simulink library "dspmtrx3"  (Simulink 8.0)
settings: Solver=ode45  SolverMode=SingleTasking  StartTime=0.0  StopTime=10.0  RelTol=1e-3
values from neighbouring files (symbols this model uses):
  a = ver('dsp')    [aboutdspsystbx.m]    (also in dsparch3Transform.m = localGetVal(inData.InstanceData, 'den', '1'); dspddes3Transform.m = sprintf('getYuleWalkerIIRFilterDesignOutput(; dspfdes.m = []; dsprprim.m = a-Mi)
  D = D + B    [rebuffer_delay.m]
undefined symbols (not defined in the file or in its folder): Floor
libraries: dspmtrx3 x5, dspsolvers x3, dspsigattribs x2, dspobslib x1, dspstat3 x1, dspfactors x1
(part 1 of 2)
settings Model: RequirementInfo=9  FPTRunName=Active  Creator=szlotkin  LastModifiedBy=lij  CovMetricSettings=d  ExtModeAutoUpdateStatusClock=off
settings Model: ForwardingTableString=|
  | ||__slOldName__||dspmtrx3/Matrix
  | Sum||__slNewName__||dspobslib/Matrix
  | Sum||__slOldName__||dspmtrx3/Matrix
  | Scaling||__slNewName__||dspmtrx3/Array-Vector
  | Multiply

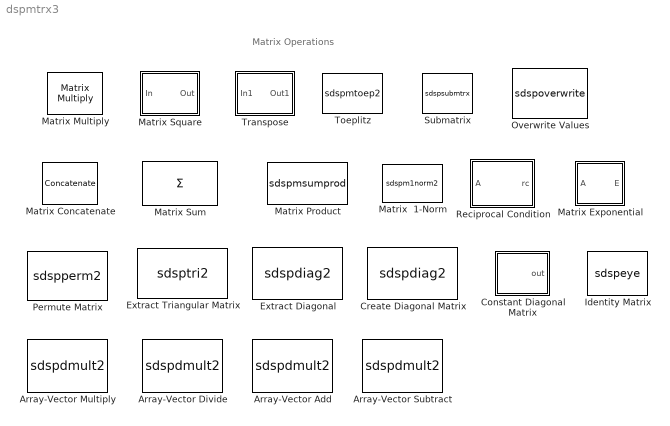
== system dspmtrx3 ==
  note: Matrix Operations
  Array-Vector Add : S-Function  DialogController=dspDDGCreate  DialogControllerArgs=DataTag0  FunctionName=sdspdmult2  Parameters=3,Dimension,V_Source,V_VectFromMask,firstCoeffMin,firstCoeffMax,outputMin,outputMax,dtInfo.firstCoeffMode,dtInfo.firstCoeffWordLength,dtInfo.firstCoeffFracLength,5,0,0,dtInfo.accumMode,dtInfo.accumWordLength,dtInfo.accumFracLength,dtInfo.outputMode,dtInfo.outputWordLength,dtInfo.outputFracLength,dtInfo.roundingMode,dtInfo.overflowMode  EnableBusSupport=off  mask(Array-Vector Add){Dimension=1, V_Source=Input port, V_VectFromMask=[0.5 0.25], additionalParams=off, allowOverrides=on, firstCoeffMode=Same word length as input, firstCoeffSignedness=Auto, firstCoeffWordLength=16, firstCoeffFracLength=15, firstCoeffDataTypeStr=Inherit: Same word length as input, firstCoeffLastDataTypeStr=Inherit: Same word length as input, firstCoeffMin=[], firstCoeffMax=[], outputMode=Same as accumulator, outputSignedness=Auto, outputWordLength=16, outputFracLength=15, outputDataTypeStr=Inherit: Same as accumulator, outputLastDataTypeStr=Inherit: Same as accumulator, outputMin=[], outputMax=[], accumMode=Inherit via internal rule, accumSignedness=Auto, accumWordLength=32, accumFracLength=30, accumDataTypeStr=Inherit: Inherit via internal rule, accumLastDataTypeStr=Inherit: Inherit via internal rule, prodOutputMode=Inherit via internal rule, prodOutputSignedness=Auto, prodOutputWordLength=32, prodOutputFracLength=30, roundingMode=Floor, overflowMode=off, LockScale=off}
      mask prompts: Dimension "Add along dimension:"; V_Source "Vector (V) source:"; V_VectFromMask "Vector (V):"; additionalParams "------- Show additional parameters -------"; allowOverrides "Allow overrides from DSP Fixed-Point Attributes blocks"; firstCoeffMode "Fixed-point scaling vector attributes:"; firstCoeffSignedness "Scaling vector elements signedness:"; firstCoeffWordLength "Scaling vector elements word length:"; firstCoeffFracLength "Scaling vector elements fraction length:"; firstCoeffDataTypeStr "Vector (V) data type string:"; firstCoeffLastDataTypeStr "Last vector (V) data type string:"; firstCoeffMin "Vector (V) minimum:"; firstCoeffMax "Vector (V) maximum:"; outputMode "Fixed-point output attributes:"; outputSignedness "Output signedness:"; outputWordLength "Output word length:"; outputFracLength "Output fraction length:"; outputDataTypeStr "Output data type string:"; outputLastDataTypeStr "Last output data type string:"; outputMin "Output minimum:"; outputMax "Output maximum:"; accumMode "Fixed-point accumulator attributes:"; accumSignedness "Accumulator signedness:"; accumWordLength "Accumulator word length"; accumFracLength "Accumulator fraction length:"; accumDataTypeStr "Accum data type string:"; accumLastDataTypeStr "Last accum data type string:"; prodOutputMode "Fixed-point product output attributes:"; prodOutputSignedness "Product output signedness:"; prodOutputWordLength "Product output word length:"; prodOutputFracLength "Product output fraction length:"; roundingMode "Round integer calculations toward:"; overflowMode "Saturate on integer overflow"; LockScale "Lock scaling"
      mask help: Add the input array A to the elements of vector V along the specified dimension. Note that unoriented input signals are treated as oriented column vectors. The output of this block is always oriented.
      mask init:
      | blkh   = gcbh;
      | dtRows = dspblkGetArrayVectorAddSubDTRowInfo();
      | dtInfo = dspGetUDTFixptDataTypeInfo(blkh, dtRows, true);
      mask Help: eval('blocksethelp');
      mask StyleString: edit,popup(Input port|Dialog parameter),edit,checkbox,checkbox,popup(Same word length as input|Specify word length|Binary point scaling|Slope and bias scaling|User-defined),popup(Auto|Signed),edit,edit,unidt({a=10|12|13|3}{i=Inherit: Same word length as input}{s=UDTBinaryPointMode}{g=UDTSignedSign}),edit,min,max,popup(Same as accumulator|Same as first input|Binary point scaling|Slope and bias scaling|User-defined),popup(Auto|Signed),edit,edit,unidt({a=18|20|21|}{i=Inherit: Same as first input|Inherit: Same as accumulator}{s=UDTBinaryPointMode}{g=UDTSignedSign|UDTInheritSign}),edit,min,max,popup(Inherit via internal rule|Same as first input|Binary point scaling|Slope and bias scaling|User-defined),popup(Auto|Signed),edit,edit,unidt({a=26|||}{i=Inherit: Inherit via internal rule|Inherit: Same as first input}{s=UDTBinaryPointMode}{g=UDTSignedSign|UDTInheritSign}),edit,popup(Inherit via internal rule|Same as first input|Binary point scaling|Slope and bias scaling|User-defined),popup(Auto|Signed),edit,edit,popup(Ceiling|Convergent|Floor|Nearest|Round|Simplest|Zero),checkbox,checkbox
      mask Display:
      | inp1_index = 1;
      | inp1_label = 'A';
      | if (V_Source == 1),
      |   inp2_index = 2;
      |   inp2_label = 'V';
      | else
      |   inp2_index = 1;
      |   inp2_label = 'A';
      | end
      | 
      | port_label('input',inp1_index,inp1_label);
      | port_label('input',inp2_index,inp2_label);
      | disp('Array-Vector\nAdd');
  Array-Vector Divide : S-Function  DialogController=dspDDGCreate  DialogControllerArgs=DataTag1  FunctionName=sdspdmult2  Parameters=2,Dimension,V_Source,V_VectFromMask,firstCoeffMin,firstCoeffMax,outputMin,outputMax,dtInfo.firstCoeffMode,dtInfo.firstCoeffWordLength,dtInfo.firstCoeffFracLength,5,0,0,5,0,0,dtInfo.outputMode,dtInfo.outputWordLength,dtInfo.outputFracLength,dtInfo.roundingMode,dtInfo.overflowMode  EnableBusSupport=off  mask(Array-Vector Divide){Dimension=1, V_Source=Input port, V_VectFromMask=[0.5 0.25], additionalParams=off, allowOverrides=on, firstCoeffMode=Same word length as input, firstCoeffSignedness=Auto, firstCoeffWordLength=16, firstCoeffFracLength=15, firstCoeffDataTypeStr=Inherit: Same word length as input, firstCoeffLastDataTypeStr=Inherit: Same word length as input, firstCoeffMin=[], firstCoeffMax=[], outputMode=Same as first input, outputSignedness=Auto, outputWordLength=16, outputFracLength=15, outputDataTypeStr=Inherit: Same as first input, outputLastDataTypeStr=Inherit: Same as first input, outputMin=[], outputMax=[], accumMode=Inherit via internal rule, accumSignedness=Auto, accumWordLength=32, accumFracLength=30, prodOutputMode=Inherit via internal rule, prodOutputSignedness=Auto, prodOutputWordLength=32, prodOutputFracLength=30, roundingMode=Floor, overflowMode=off, LockScale=off}
      mask prompts: Dimension "Divide along dimension:"; V_Source "Vector (V) source:"; V_VectFromMask "Vector (V):"; additionalParams "------- Show additional parameters -------"; allowOverrides "Allow overrides from DSP Fixed-Point Attributes blocks"; firstCoeffMode "Fixed-point scaling vector attributes:"; firstCoeffSignedness "Scaling vector elements signedness:"; firstCoeffWordLength "Scaling vector elements word length:"; firstCoeffFracLength "Scaling vector elements fraction length:"; firstCoeffDataTypeStr "Vector (V) data type string:"; firstCoeffLastDataTypeStr "Last vector (V) data type string:"; firstCoeffMin "Vector (V) minimum:"; firstCoeffMax "Vector (V) maximum:"; outputMode "Fixed-point output attributes:"; outputSignedness "Output signedness:"; outputWordLength "Output word length:"; outputFracLength "Output fraction length:"; outputDataTypeStr "Output data type string:"; outputLastDataTypeStr "Last output data type string:"; outputMin "Output minimum:"; outputMax "Output maximum:"; accumMode "Fixed-point accumulator attributes:"; accumSignedness "Accumulator signedness:"; accumWordLength "Accumulator word length"; accumFracLength "Accumulator fraction length:"; prodOutputMode "Fixed-point product output attributes:"; prodOutputSignedness "Product output signedness:"; prodOutputWordLength "Product output word length:"; prodOutputFracLength "Product output fraction length:"; roundingMode "Round integer calculations toward:"; overflowMode "Saturate on integer overflow"; LockScale "Lock scaling"
      mask help: Divide the input array A by the elements of vector V along the specified dimension. In the two-dimensional case, this is equivalent to dividing a full matrix (A) by a diagonal (V). Note that unoriented input signals are treated as oriented column vectors. The output of this block is always oriented.
      mask init:
      | blkh   = gcbh;
      | dtRows = dspblkGetArrayVectorDivDTRowInfo();
      | dtInfo = dspGetUDTFixptDataTypeInfo(blkh, dtRows, true);
      mask Help: eval('blocksethelp');
      mask StyleString: edit,popup(Input port|Dialog parameter),edit,checkbox,checkbox,popup(Same word length as input|Specify word length|Binary point scaling|Slope and bias scaling|User-defined),popup(Auto|Signed),edit,edit,unidt({a=10|12|13|3}{i=Inherit: Same word length as input}{s=UDTBinaryPointMode}{g=UDTSignedSign}),edit,min,max,popup(Same as first input|Binary point scaling|Slope and bias scaling|User-defined),popup(Auto|Signed),edit,edit,unidt({a=18|20|21|}{i=Inherit: Same as first input}{s=UDTBinaryPointMode}{g=UDTSignedSign|UDTInheritSign}),edit,min,max,popup(Inherit via internal rule|Same as product output|Same as first input|Binary point scaling|Slope and bias scaling|User-defined),popup(Auto|Signed),edit,edit,popup(Inherit via internal rule|Same as first input|Binary point scaling|Slope and bias scaling|User-defined),popup(Auto|Signed),edit,edit,popup(Ceiling|Convergent|Floor|Nearest|Round|Simplest|Zero),checkbox,checkbox
      mask Display:
      | inp1_index = 1;
      | inp1_label = 'A';
      | if (V_Source == 1),
      |   inp2_index = 2;
      |   inp2_label = 'V';
      | else
      |   inp2_index = 1;
      |   inp2_label = 'A';
      | end
      | 
      | port_label('input',inp1_index,inp1_label);
      | port_label('input',inp2_index,inp2_label);
      | disp('Array-Vector\nDivide');
  Array-Vector Multiply : S-Function  DialogController=dspDDGCreate  DialogControllerArgs=DataTag2  FunctionName=sdspdmult2  Parameters=1,Dimension,V_Source,V_VectFromMask,firstCoeffMin,firstCoeffMax,outputMin,outputMax,dtInfo.firstCoeffMode,dtInfo.firstCoeffWordLength,dtInfo.firstCoeffFracLength,dtInfo.prodOutputMode,dtInfo.prodOutputWordLength,dtInfo.prodOutputFracLength,dtInfo.accumMode,dtInfo.accumWordLength,dtInfo.accumFracLength,dtInfo.outputMode,dtInfo.outputWordLength,dtInfo.outputFracLength,dtInfo.roundingMode,dtInfo.overflowMode  EnableBusSupport=off  mask(Array-Vector Multiply){mode=Mute, saveAsFlag=0, Dimension=2, V_Source=Input port, V_VectFromMask=[0.5 0.25], additionalParams=off, allowOverrides=on, firstCoeffMode=Same word length as input, firstCoeffSignedness=Auto, firstCoeffWordLength=16, firstCoeffFracLength=15, firstCoeffDataTypeStr=Inherit: Same word length as input, firstCoeffLastDataTypeStr=Inherit: Same word length as input, firstCoeffMin=[], firstCoeffMax=[], outputMode=Same as product output, outputSignedness=Auto, outputWordLength=16, outputFracLength=15, outputDataTypeStr=Inherit: Same as product output, outputLastDataTypeStr=Inherit: Same as product output, outputMin=[], outputMax=[], accumMode=Inherit via internal rule, accumSignedness=Auto, accumWordLength=32, accumFracLength=30, accumDataTypeStr=Inherit: Inherit via internal rule, accumLastDataTypeStr=Inherit: Inherit via internal rule, prodOutputMode=Inherit via internal rule, prodOutputSignedness=Auto, prodOutputWordLength=32, prodOutputFracLength=30, prodOutputDataTypeStr=Inherit: Inherit via internal rule, prodOutputLastDataTypeStr=Inherit: Inherit via internal rule, roundingMode=Floor, overflowMode=off, LockScale=off}
      mask prompts: saveAsFlag "Save_as flag:"; Dimension "Multiply along dimension:"; V_Source "Vector (V) source:"; V_VectFromMask "Vector (V):"; additionalParams "------- Show additional parameters -------"; allowOverrides "Allow overrides from DSP Fixed-Point Attributes blocks"; firstCoeffMode "Fixed-point scaling vector attributes:"; firstCoeffSignedness "Scaling vector elements signedness:"; firstCoeffWordLength "Scaling vector elements word length:"; firstCoeffFracLength "Scaling vector elements fraction length:"; firstCoeffDataTypeStr "Vector (V) data type string:"; firstCoeffLastDataTypeStr "Last vector (V) data type string:"; firstCoeffMin "Last vector (V) minimum:"; firstCoeffMax "Last vector (V) maximum:"; outputMode "Fixed-point output attributes:"; outputSignedness "Output signedness:"; outputWordLength "Output word length:"; outputFracLength "Output fraction length:"; outputDataTypeStr "Output data type string:"; outputLastDataTypeStr "Last output data type string:"; outputMin "Output minimum:"; outputMax "Output maximum:"; accumMode "Fixed-point accumulator attributes:"; accumSignedness "Accumulator signedness:"; accumWordLength "Accumulator word length"; accumFracLength "Accumulator fraction length:"; accumDataTypeStr "Accum data type string:"; accumLastDataTypeStr "Last accum data type string:"; prodOutputMode "Fixed-point product output attributes:"; prodOutputSignedness "Product output signedness:"; prodOutputWordLength "Product output word length:"; prodOutputFracLength "Product output fraction length:"; prodOutputDataTypeStr "ProdOutput data type string:"; prodOutputLastDataTypeStr "Last prodOutput data type string:"; roundingMode "Round integer calculations toward:"; overflowMode "Saturate on integer overflow"; LockScale "Lock scaling"
      mask help: Multiply the input array A by the elements of vector V along the specified dimension. In the two-dimensional case, this is equivalent to multiplying a full matrix (A) by a diagonal (V). Note that unoriented input signals are treated as oriented column vectors. The output of this block is always oriented.
      mask init:
      | blkh = gcbh;
      | m    = get_param(blkh, 'mode');
      | if (~strcmp(m, 'Mute'))
      |     if (saveAsFlag == 0)
      |         if strcmp(m,'Scale rows (D*A)')
      |             set_param(blkh, 'Dimension', '1', 'mode', 'Mute');
      |         elseif strcmp(m,'Scale columns (A*D)')
      |             set_param(blkh, 'Dimension', '2', 'mode', 'Mute');
      |         end
      |     end
      | end
      | dtRows = dspblkGetArrayVectorMpyDTRowInfo();
      | dtInfo = dspGetUDTFixptDataTypeInfo(blkh, dtRows, true);
      mask Help: eval('blocksethelp');
      mask StyleString: popup(Scale rows (D*A)|Scale columns (A*D)|Mute),edit,edit,popup(Input port|Dialog parameter),edit,checkbox,checkbox,popup(Same word length as input|Specify word length|Binary point scaling|Slope and bias scaling|User-defined),popup(Auto|Signed),edit,edit,unidt({a=12|14|15|5}{i=Inherit: Same word length as input}{s=UDTBinaryPointMode}{g=UDTSignedSign}),edit,min,max,popup(Same as product output|Same as first input|Binary point scaling|Slope and bias scaling|User-defined),popup(Auto|Signed),edit,edit,unidt({a=20|22|23|}{i=Inherit: Same as first input|Inherit: Same as product output}{s=UDTBinaryPointMode}{g=UDTSignedSign|UDTInheritSign}),edit,min,max,popup(Inherit via internal rule|Same as product output|Same as first input|Binary point scaling|Slope and bias scaling|User-defined),popup(Auto|Signed),edit,edit,unidt({a=28|||}{i=Inherit: Inherit via internal rule|Inherit: Same as first input|Inherit: Same as product output}{s=UDTBinaryPointMode}{g=UDTSignedSign|UDTInheritSign}),edit,popup(Inherit via internal rule|Same as first input|Binary point scaling|Slope and bias scaling|User-defined),popup(Auto|Signed),edit,edit,unidt({a=34|||}{i=Inherit: Inherit via internal rule|Inherit: Same as first input}{s=UDTBinaryPointMode}{g=UDTSignedSign|UDTInheritSign}),edit,popup(Ceiling|Convergent|Floor|Nearest|Round|Simplest|Zero),checkbox,checkbox
      mask Display:
      | inp1_index = 1;
      | inp1_label = 'A';
      | if (V_Source == 1),
      |   inp2_index = 2;
      |   inp2_label = 'V';
      | else
      |   inp2_index = 1;
      |   inp2_label = 'A';
      | end
      | 
      | port_label('input',inp1_index,inp1_label);
      | port_label('input',inp2_index,inp2_label);
      | disp('Array-Vector\nMultiply');
  Array-Vector Subtract : S-Function  DialogController=dspDDGCreate  DialogControllerArgs=DataTag3  FunctionName=sdspdmult2  Parameters=4,Dimension,V_Source,V_VectFromMask,firstCoeffMin,firstCoeffMax,outputMin,outputMax,dtInfo.firstCoeffMode,dtInfo.firstCoeffWordLength,dtInfo.firstCoeffFracLength,5,0,0,dtInfo.accumMode,dtInfo.accumWordLength,dtInfo.accumFracLength,dtInfo.outputMode,dtInfo.outputWordLength,dtInfo.outputFracLength,dtInfo.roundingMode,dtInfo.overflowMode  EnableBusSupport=off  mask(Array-Vector Subtract){Dimension=1, V_Source=Input port, V_VectFromMask=[0.5 0.25], additionalParams=off, allowOverrides=on, firstCoeffMode=Same word length as input, firstCoeffSignedness=Auto, firstCoeffWordLength=16, firstCoeffFracLength=15, firstCoeffDataTypeStr=Inherit: Same word length as input, firstCoeffLastDataTypeStr=Inherit: Same word length as input, firstCoeffMin=[], firstCoeffMax=[], outputMode=Same as accumulator, outputSignedness=Auto, outputWordLength=16, outputFracLength=15, outputDataTypeStr=Inherit: Same as accumulator, outputLastDataTypeStr=Inherit: Same as accumulator, outputMin=[], outputMax=[], accumMode=Inherit via internal rule, accumSignedness=Auto, accumWordLength=32, accumFracLength=30, accumDataTypeStr=Inherit: Inherit via internal rule, accumLastDataTypeStr=Inherit: Inherit via internal rule, prodOutputMode=Inherit via internal rule, prodOutputSignedness=Auto, prodOutputWordLength=32, prodOutputFracLength=30, roundingMode=Floor, overflowMode=off, LockScale=off}
      mask prompts: Dimension "Subtract along dimension:"; V_Source "Vector (V) source:"; V_VectFromMask "Vector (V):"; additionalParams "------- Show additional parameters -------"; allowOverrides "Allow overrides from DSP Fixed-Point Attributes blocks"; firstCoeffMode "Fixed-point scaling vector attributes:"; firstCoeffSignedness "Scaling vector elements signedness:"; firstCoeffWordLength "Scaling vector elements word length:"; firstCoeffFracLength "Scaling vector elements fraction length:"; firstCoeffDataTypeStr "Vector (V) data type string:"; firstCoeffLastDataTypeStr "Last vector (V) data type string:"; firstCoeffMin "Vector (V) minimum:"; firstCoeffMax "Vector (V) maximum:"; outputMode "Fixed-point output attributes:"; outputSignedness "Output signedness:"; outputWordLength "Output word length:"; outputFracLength "Output fraction length:"; outputDataTypeStr "Output data type string:"; outputLastDataTypeStr "Last output data type string:"; outputMin "Output minimum:"; outputMax "Output maximum:"; accumMode "Fixed-point accumulator attributes:"; accumSignedness "Accumulator signedness:"; accumWordLength "Accumulator word length"; accumFracLength "Accumulator fraction length:"; accumDataTypeStr "Accum data type string:"; accumLastDataTypeStr "Last accum data type string:"; prodOutputMode "Fixed-point product output attributes:"; prodOutputSignedness "Product output signedness:"; prodOutputWordLength "Product output word length:"; prodOutputFracLength "Product output fraction length:"; roundingMode "Round integer calculations toward:"; overflowMode "Saturate on integer overflow"; LockScale "Lock scaling"
      mask help: Subtract the elements of vector V from input array A along the specified dimension. Note that unoriented input signals are treated as oriented column vectors. The output of this block is always oriented.
      mask init:
      | blkh   = gcbh;
      | dtRows = dspblkGetArrayVectorAddSubDTRowInfo();
      | dtInfo = dspGetUDTFixptDataTypeInfo(blkh, dtRows, true);
      mask Help: eval('blocksethelp');
      mask StyleString: edit,popup(Input port|Dialog parameter),edit,checkbox,checkbox,popup(Same word length as input|Specify word length|Binary point scaling|Slope and bias scaling|User-defined),popup(Auto|Signed),edit,edit,unidt({a=10|12|13|3}{i=Inherit: Same word length as input}{s=UDTBinaryPointMode}{g=UDTSignedSign}),edit,min,max,popup(Same as accumulator|Same as first input|Binary point scaling|Slope and bias scaling|User-defined),popup(Auto|Signed),edit,edit,unidt({a=18|20|21|}{i=Inherit: Same as first input|Inherit: Same as accumulator}{s=UDTBinaryPointMode}{g=UDTSignedSign|UDTInheritSign}),edit,min,max,popup(Inherit via internal rule|Same as first input|Binary point scaling|Slope and bias scaling|User-defined),popup(Auto|Signed),edit,edit,unidt({a=26|||}{i=Inherit: Inherit via internal rule|Inherit: Same as first input}{s=UDTBinaryPointMode}{g=UDTSignedSign|UDTInheritSign}),edit,popup(Inherit via internal rule|Same as first input|Binary point scaling|Slope and bias scaling|User-defined),popup(Auto|Signed),edit,edit,popup(Ceiling|Convergent|Floor|Nearest|Round|Simplest|Zero),checkbox,checkbox
      mask Display:
      | inp1_index = 1;
      | inp1_label = 'A';
      | if (V_Source == 1),
      |   inp2_index = 2;
      |   inp2_label = 'V';
      | else
      |   inp2_index = 1;
      |   inp2_label = 'A';
      | end
      | 
      | port_label('input',inp1_index,inp1_label);
      | port_label('input',inp2_index,inp2_label);
      | disp('Array-Vector\nSubtract');
  Constant Diagonal Matrix : Subsystem  mask(Constant Diagonal Matrix){q=ones(1,3), frame=off, additionalParams=off, allowOverrides=on, dataType=Inherit from 'Constant(s) along diagonal', isSigned=on, wordLen=16, udDataType=sfix(16), fracBitsMode=Best precision, numFracBits=15}
      mask prompts: q "Constant(s) along diagonal:"; frame "Frame-based output"; additionalParams "------- Show additional parameters --------"; allowOverrides "Allow overrides by DSP Fixed-Point Attributes blocks"; dataType "Output data type:"; isSigned "Signed"; wordLen "Word length:"; udDataType "User-defined data type:"; fracBitsMode "Set fraction length in output to:"; numFracBits "Fraction length:"
      mask help: Generate a diagonal matrix having elements specified by a vector constant.
      mask init:
      | [a,x,y] = dspblkconstdiag('icon',q);
      | dspblkconstdiag('init');
      mask Help: eval('blocksethelp');
      mask StyleString: edit,checkbox,checkbox,checkbox,popup(double|single|int8|uint8|int16|uint16|int32|uint32|boolean|Fixed-point|User-defined|Inherit from 'Constant(s) along diagonal'|Inherit via back propagation),checkbox,edit,edit,popup(Best precision|User-defined),edit
      mask CallbackString: ||||dspblkconstdiag;|||dspblkconstdiag;|dspblkconstdiag;|
      mask TabNameString: Main,Main,Main,Main,Data Types,Data Types,Data Types,Data Types,Data Types,Data Types
      mask Display: plot(x,y)
  Create Diagonal Matrix : S-Function  FunctionName=sdspdiag2  Parameters=mode  EnableBusSupport=off  mask(Create Diagonal Matrix){}
      mask help: Convert a vector of diagonal elements to a full matrix.
      mask init:
      | mode = 1;
      | x = [.58 .87 .87 .58 .58 NaN 0.45 0.12 NaN 0.525 0.525 0.475 0.475 0.525 0.525 0.565 0.525 ];
      | y = [ 0.2 0.2 0.8 0.8 0.2 NaN 0.2 0.8 NaN 0.435 0.475 0.475 0.525 0.525 0.565 0.5 0.435 ];
      mask Help: eval('blocksethelp');
      mask Display:
      | plot(x,y);
      | port_label('input',1,'D');
      | port_label('output',1,'A');
  Extract Diagonal : S-Function  FunctionName=sdspdiag2  Parameters=mode  EnableBusSupport=off  mask(Extract Diagonal){}
      mask help: Extract the main diagonal of a full matrix.
      mask init:
      | mode = 2;
      | x = [.58 .87 NaN 0.12 0.45 0.45 0.12 0.12 NaN 0.525 0.525 0.475 0.475 0.525 0.525 0.565 0.525 ];
      | y = [ 0.8 0.2 NaN 0.2 0.2 0.8 0.8 0.2 NaN 0.435 0.475 0.475 0.525 0.525 0.565 0.5 0.435 ];
      mask Help: eval('blocksethelp');
      mask Display:
      | plot(x,y);
      | port_label('input',1,'A');
      | port_label('output',1,'D');
  Extract Triangular Matrix : S-Function  FunctionName=sdsptri2  Parameters=fcn  EnableBusSupport=off  mask(Extract Triangular Matrix){fcn=Upper}
      mask prompts: fcn "Extract:"
      mask help: Extract upper or lower triangular part of input matrix.
      mask init:
      | [s,x,y] = dspblktri(fcn);
      mask Help: eval('blocksethelp');
      mask StyleString: popup(Upper|Lower)
      mask Display:
      | plot(x,y);
      | port_label('input',1,'A');
      | port_label('output',1,s);
  Identity Matrix : S-Function  FunctionName=sdspeye  Parameters=Inherit,N,Ts,isCustomFloat,fxpIsSigned,dTypeID,fxpWordLength,fxpFracLength,1  EnableBusSupport=off  mask(Identity Matrix){Inherit=off, N=5, Ts=1, additionalParams=off, allowOverrides=on, dataType=double, isSigned=on, wordLen=16, udDataType=sfix(16), fracBitsMode=Best precision, numFracBits=15, OutDataTypeStr=double, LastOutDataTypeStr=double}
      mask prompts: Inherit "Inherit output port attributes from input port"; N "Matrix size:"; Ts "Sample time:"; additionalParams "------- Show additional parameters --------"; allowOverrides "Allow overrides by DSP Fixed-Point Attributes blocks"; dataType "Output data type:"; isSigned "Signed"; wordLen "Word length:"; udDataType "User-defined data type (e.g. sfix(16), float('single')):"; fracBitsMode "Set fraction length in output to:"; numFracBits "Fraction length:"; OutDataTypeStr "Output data type:"; LastOutDataTypeStr "Last output data type:"
      mask help: Output an identity matrix. If the matrix size entered is a scalar, then the output will be a square (symmetric) identity matrix with the number of rows and columns both equal to the specified value. If the matrix size entered is a two-element vector [M N], then the output will be an asymmetric matrix with the number of rows equal to M, the number of columns equal to N, ones down the diagonal, and zeros elsewhere. This matches the syntax of the MATLAB function eye(N) and eye(M,N), respectively.
      mask init:
      | isCustomFloat =  0; % nice default
      | fxpIsSigned   =  1; % nice default
      | fxpWordLength =  8; % nice default
      | fxpFracLength =  0; % nice default
      | if Inherit
      |     dTypeID   = -3; % SAME_AS_INPUT
      | else
      |     dtRows            = dspblkGetDiscreteImpulseDTRowInfo();
      |     [dtInfo, dTypeID] = dspblkUDTMapperOutDType(gcbh, dtRows{1}, 'dataType', 1.0);
      |     isCustomFloat     = dtInfo.DataTypeIsCustomFloat;
      |     if ~isCustomFloat
      |         fxpIsSigned   = dtInfo.DataTypeIsSigned;
      |         fxpWordLength = dtInfo.DataTypeWordLength;
      |         fxpFracLength = dtInfo.DataTypeFracOrMantBits;
      |     end
      | end
      mask Help: eval('blocksethelp');
      mask StyleString: checkbox,edit,edit,checkbox,checkbox,popup(double|single|int8|uint8|int16|uint16|int32|uint32|boolean|Fixed-point|User-defined|Inherit via back propagation),checkbox,edit,edit,popup(Best precision|User-defined),edit,unidt({a=12|||}{i=Inherit: Inherit via back propagation}{b=double|single|int8|uint8|int16|uint16|int32|uint32|boolean}{s=UDTBinaryPointMode|UDTBestPrecisionMode}{g=UDTSignedSign|UDTUnsignedSign}),edit
      mask CallbackString: dspblkeye||||||||||||
      mask TabNameString: Main,Main,Main,Data Types,Data Types,Data Types,Data Types,Data Types,Data Types,Data Types,Data Types,Data Types,Data Types
      mask Display:
      | if Inherit
      |     disp('eye( )');
      | else
      |     disp(['eye(' , num2str(get_param(gcbh, 'N')), ')']);
      | end
  Matrix Concatenate : Concatenate  Mode=Multidimensional array  ConcatenateDimension=2
  Matrix Exponential : Subsystem
      mask Type: Matrix Exponential
      mask Description: Compute the matrix exponential, using a scaling and squaring algorithm with a Pade approximation.  Matrix must be square.
      mask Help: eval('blocksethelp');
      mask Display: disp('expm')
  Matrix Product : S-Function  DialogController=dspDDGCreate  DialogControllerArgs=DataTag4  FunctionName=sdspmsumprod  Parameters=Dim,2,outputMin,outputMax,dtInfo.interProdMode,dtInfo.interProdWordLength,dtInfo.interProdFracLength,dtInfo.prodOutputMode,dtInfo.prodOutputWordLength,dtInfo.prodOutputFracLength,dtInfo.accumMode,dtInfo.accumWordLength,dtInfo.accumFracLength,dtInfo.outputMode,dtInfo.outputWordLength,dtInfo.outputFracLength,dtInfo.roundingMode,dtInfo.overflowMode  EnableBusSupport=off  mask(Matrix Product){Dim=Columns, additionalParams=off, allowOverrides=on, outputMode=Same as product output, outputWordLength=16, outputFracLength=15, outputDataTypeStr=Inherit: Same as product output, outputLastDataTypeStr=Inherit: Same as product output, outputMin=[], outputMax=[], accumMode=Inherit via internal rule, accumWordLength=32, accumFracLength=30, accumDataTypeStr=Inherit: Inherit via internal rule, accumLastDataTypeStr=Inherit: Inherit via internal rule, prodOutputMode=Inherit via internal rule, prodOutputWordLength=32, prodOutputFracLength=30, prodOutputDataTypeStr=Inherit: Inherit via internal rule, prodOutputLastDataTypeStr=Inherit: Inherit via internal rule, interProdMode=Same as input, interProdWordLength=16, interProdFracLength=15, interProdDataTypeStr=Inherit: Same as input, interProdLastDataTypeStr=Inherit: Same as input, roundingMode=Floor, overflowMode=off, LockScale=off}
      mask prompts: Dim "Multiply over:"; additionalParams "------- Show additional parameters -------"; allowOverrides "Allow overrides from DSP Fixed-Point Attributes blocks"; outputMode "Fixed-point output attributes:"; outputWordLength "Output word length:"; outputFracLength "Output fraction length:"; outputDataTypeStr "Output data type string:"; outputLastDataTypeStr "Last output data type string:"; outputMin "Output minimum:"; outputMax "Output maximum:"; accumMode "Fixed-point accumulator attributes:"; accumWordLength "Accumulator word length:"; accumFracLength "Accumulator fraction length:"; accumDataTypeStr "Accum data type string:"; accumLastDataTypeStr "Last accum data type string:"; prodOutputMode "Fixed-point product output attributes:"; prodOutputWordLength "Product output word length:"; prodOutputFracLength "Product output fraction length:"; prodOutputDataTypeStr "ProdOutput data type string:"; prodOutputLastDataTypeStr "Last prodOutput data type string:"; interProdMode "Fixed-point intermediate product attributes:"; interProdWordLength "Intermediate product word length:"; interProdFracLength "Intermediate product fraction length:"; interProdDataTypeStr "Intermediate product data type string:"; interProdLastDataTypeStr "Last intermediate product data type string:"; roundingMode "Round integer calculations toward:"; overflowMode "Saturate on integer overflow"; LockScale "Lock scaling"
      mask help: Multiply the elements of a matrix along its rows, its columns, or over all its elements. Note that 1-D input signals produce a single scalar output equal to the product of the individual elements.
      mask init:
      | blkh   = gcbh;
      | dtRows = dspblkGetMtrxProdDTRowInfo();
      | dtInfo = dspGetUDTFixptDataTypeInfo(blkh, dtRows, true);
      mask Help: eval('blocksethelp');
      mask StyleString: popup(Rows|Columns|Entire input),checkbox,checkbox,popup(Same as product output|Same as input|Binary point scaling|Slope and bias scaling|User-defined),edit,edit,unidt({a=7|9|10|}{i=Inherit: Same as input|Inherit: Same as product output}{s=UDTBinaryPointMode}{g=UDTInheritSign}),edit,min,max,popup(Inherit via internal rule|Same as product output|Same as input|Binary point scaling|Slope and bias scaling|User-defined),edit,edit,unidt({a=14|||}{i=Inherit: Inherit via internal rule|Inherit: Same as input|Inherit: Same as product output}{s=UDTBinaryPointMode}{g=UDTInheritSign}),edit,popup(Inherit via internal rule|Same as input|Binary point scaling|Slope and bias scaling|User-defined),edit,edit,unidt({a=19|||}{i=Inherit: Inherit via internal rule|Inherit: Same as input}{s=UDTBinaryPointMode}{g=UDTInheritSign}),edit,popup(Same as input|Binary point scaling|Slope and bias scaling|User-defined),edit,edit,unidt({a=24|||}{i=Inherit: Same as input}{s=UDTBinaryPointMode}{g=UDTInheritSign}),edit,popup(Ceiling|Convergent|Floor|Nearest|Round|Simplest|Zero),checkbox,checkbox
      mask Display:
      | if (Dim==1), str='Row\nProduct';
      | elseif (Dim==2), str='Column\nProduct';
      | else str='Product of\nAll Elements';
      | end
      | disp(str);
  Matrix Square : Subsystem  mask(Matrix Square){OutMin=[], OutMax=[], OutDataTypeStr=Inherit: Inherit via internal rule, LockScale=off, RndMeth=Floor, SaturateOnIntegerOverflow=off}
      mask prompts: OutMin "Output minimum:"; OutMax "Output maximum:"; OutDataTypeStr "Output data type:"; LockScale "Lock output data type setting against changes by the fixed-point tools"; RndMeth "Integer rounding mode:"; SaturateOnIntegerOverflow "Saturate on integer overflow"
      mask help: Compute the matrix square, U' * U. Hermitian transpose is performed for complex inputs. [Mx1] and [1xN] input matrices may be used to compute efficient outer and inner products, respectively.
      mask init:
      | mtxsqName = gcb;
      | trnspName = sprintf('%s/Math\nFunction', mtxsqName);
      | prdctName = sprintf('%s/Product', mtxsqName);
      | % Set matrix transpose block parameters
      | set_param(trnspName, 'SaturateOnIntegerOverflow', SaturateOnIntegerOverflow);
      | % Set matrix product block parameters
      | set_param(prdctName, 'SaturateOnIntegerOverflow', SaturateOnIntegerOverflow);
      | switch RndMeth
      |     case 1
      |         set_param(prdctName, 'RndMeth', 'Ceiling');
      |     case 2
      |         set_param(prdctName, 'RndMeth', 'Convergent');
      |     case 3
      |         set_param(prdctName, 'RndMeth', 'Floor');
      |     case 4
      |         set_param(prdctName, 'RndMeth', 'Nearest');
      |     case 5
      |         set_param(prdctName, 'RndMeth', 'Round');
      |     case 6
      |         set_param(prdctName, 'RndMeth', 'Simplest');
      |     otherwise
      |         set_param(prdctName, 'RndMeth', 'Zero');
      | end
      mask Help: eval('blocksethelp');
      mask StyleString: min,max,unidt({a=3|1|2|}{i=Inherit: Inherit via internal rule|Inherit: Inherit via back propagation|Inherit: Same as first input}{b=double|single|int8|uint8|int16|uint16|int32|uint32}{s=UDTBinaryPointMode}{g=UDTSignedSign|UDTUnsignedSign}),checkbox,popup(Ceiling|Convergent|Floor|Nearest|Round|Simplest|Zero),checkbox
      mask TabNameString: Signal Attributes,Signal Attributes,Signal Attributes,Signal Attributes,Signal Attributes,Signal Attributes
      mask Display: disp('u^Hu','texmode','on')
  Matrix Sum : Sum  Inputs=+
  Matrix  1-Norm : S-Function  DialogController=dspDDGCreate  DialogControllerArgs=DataTag5  FunctionName=sdspm1norm2  Parameters=outputMin,outputMax,dtInfo.accumMode,dtInfo.accumWordLength,dtInfo.accumFracLength,dtInfo.outputMode,dtInfo.outputWordLength,dtInfo.outputFracLength,dtInfo.roundingMode,dtInfo.overflowMode  EnableBusSupport=off  mask(Matrix 1-Norm){allowOverrides=on, outputMode=Same as accumulator, outputWordLength=16, outputFracLength=15, outputDataTypeStr=Inherit: Same as accumulator, outputLastDataTypeStr=Inherit: Same as accumulator, outputMin=[], outputMax=[], accumMode=Inherit via internal rule, accumWordLength=32, accumFracLength=30, accumDataTypeStr=Inherit: Inherit via internal rule, accumLastDataTypeStr=Inherit: Inherit via internal rule, roundingMode=Floor, overflowMode=off, LockScale=off}
      mask prompts: allowOverrides "Allow overrides from DSP Fixed-Point Attributes blocks"; outputMode "Fixed-point output attributes:"; outputWordLength "Output word length:"; outputFracLength "Output fraction length:"; outputDataTypeStr "Output data type string:"; outputLastDataTypeStr "Last output data type string:"; outputMin "Output minimum:"; outputMax "Output maximum:"; accumMode "Fixed-point accumulator attributes:"; accumWordLength "Accumulator word length:"; accumFracLength "Accumulator fraction length:"; accumDataTypeStr "Accum data type string:"; accumLastDataTypeStr "Last accum data type string:"; roundingMode "Round integer calculations toward:"; overflowMode "Saturate on integer overflow"; LockScale "Lock scaling"
      mask help: Compute the matrix 1-norm, which is the largest column sum of absolute values. Note that unoriented input signals are treated as oriented column vectors. The output of this block is always oriented.
      mask init:
      | blkh   = gcbh;
      | dtRows = dspblkGetM1NormDTRowInfo();
      | dtInfo = dspGetUDTFixptDataTypeInfo(blkh, dtRows, true);
      mask Help: eval('blocksethelp');
      mask StyleString: checkbox,popup(Same as accumulator|Same as input|Binary point scaling|Slope and bias scaling|User-defined),edit,edit,unidt({a=5|7|8|}{i=Inherit: Same as input|Inherit: Same as accumulator}{s=UDTBinaryPointMode}{g=UDTInheritSign}),edit,min,max,popup(Inherit via internal rule|Same as input|Binary point scaling|Slope and bias scaling|User-defined),edit,edit,unidt({a=12|||}{i=Inherit: Inherit via internal rule|Inherit: Same as input}{s=UDTBinaryPointMode}{g=UDTInheritSign}),edit,popup(Ceiling|Convergent|Floor|Nearest|Round|Simplest|Zero),checkbox,checkbox
      mask Display: disp('Matrix\n1-Norm')
  Matrix Multiply : Product  Multiplication=Matrix(*)
  Overwrite Values : S-Function  FunctionName=sdspoverwrite  Parameters=ColSpan, ColStartMode, ColStartIndex, ColEndMode, ColEndIndex, RowSpan, RowStartMode, RowStartIndex, RowEndMode, RowEndIndex, OverWriteDiag, ConstValue, DiagSpan, DiagStartMode, DiagStartIndex, DiagEndMode, DiagEndIndex, valFrom2ndIP  EnableBusSupport=off  mask(Overwrite Values){OverWriteDiag=Submatrix, valFrom2ndIP=Specify via dialog, ConstValue=0, RowSpan=Range of rows, RowStartMode=First, RowStartIndex=1, RowEndMode=Last, RowEndIndex=1, ColSpan=Range of columns, ColStartMode=First, ColStartIndex=1, ColEndMode=Last, ColEndIndex=1, DiagSpan=Range of elements, DiagStartMode=Index, DiagStartIndex=2, DiagEndMode=Index, DiagEndIndex=4}
      mask prompts: OverWriteDiag "Overwrite:"; valFrom2ndIP "Source of overwriting value(s):"; ConstValue "Overwrite with:"; RowSpan "Row span:"; RowStartMode "Starting row:"; RowStartIndex "Starting row index:"; RowEndMode "Ending row:"; RowEndIndex "Ending row index:"; ColSpan "Column span:"; ColStartMode "Starting column:"; ColStartIndex "Starting column index:"; ColEndMode "Ending column:"; ColEndIndex "Ending column index:"; DiagSpan "Diagonal span:"; DiagStartMode "Starting element:"; DiagStartIndex "Starting element index:"; DiagEndMode "Ending element:"; DiagEndIndex "Ending element index:"
      mask help:
      | Overwrites a selected portion of the input matrix--either a submatrix, full diagonal, or a portion of the diagonal.
      | Specify overwriting values as follows:
      |   --Matrix with the same dimensions as the submatrix
      |   --Vector with the same length as the portion of the diagonal
      |   --Scalar constant with which to replace each element in the submatrix or diagonal portion.
      |
      | Treats unoriented (1-D) input vectors as column vectors.
      mask init:
      | [x1,y1,xc,yc,xmc,ymc,xi,yi] = dspblkoverwrite('icon');
      | if valFrom2ndIP == 1
      |   i1=1;
      |   s1='';
      | else
      |   i1=2;
      |   s1='V';
      | end;
      mask Help: eval('blocksethelp');
      mask StyleString: popup(Submatrix|Diagonal),popup(Specify via dialog|Second input port),edit,popup(All rows|One row|Range of rows),popup(First|Index|Offset from last|Last|Offset from middle|Middle),edit,popup(Index|Offset from last|Last|Offset from middle|Middle),edit,popup(All columns|One column|Range of columns),popup(First|Index|Offset from last|Last|Offset from middle|Middle),edit,popup(Index|Offset from last|Last|Offset from middle|Middle),edit,popup(All elements|One element|Range of elements),popup(First|Index|Offset from last|Last|Offset from middle|Middle),edit,popup(Index|Offset from last|Last|Offset from middle|Middle),edit
      mask CallbackString: dspblkoverwrite|dspblkoverwrite||dspblkoverwrite|dspblkoverwrite||dspblkoverwrite||dspblkoverwrite|dspblkoverwrite||dspblkoverwrite||dspblkoverwrite|dspblkoverwrite||dspblkoverwrite|
      mask Display:
      | plot(x1,y1,xc,yc,xmc,ymc,xi,yi);
      | port_label('input',1,'A');
      | port_label('output',1,'B');
      | port_label('input',i1,s1);
  Permute Matrix : S-Function  FunctionName=sdspperm2  Parameters=0,1,mode,2,0,0,0,errmode,checkDims, ZeroOneIdxMode  EnableBusSupport=off  mask(Permute Matrix){mode=Columns, ZeroOneIdxMode=One-based, errmode=Clip Index, checkDims=off}
      mask prompts: mode "Permute:"; ZeroOneIdxMode "Index mode:"; errmode "Invalid permutation index:"; checkDims "Error when length of P is not equal to Permute dimension size"
      mask help: Permutes the rows or columns of a matrix or vector A, based on a vector P of integer-valued permutation indices. The indices need not be unique. When you select the Error check box, the length of vector P must be the same as the number of input rows or columns (whichever you are permuting).
      mask init:
      | modeVal = get_param(gcbh, 'mode');
      mask Help: eval('blocksethelp');
      mask StyleString: popup(Rows|Columns),popup(Zero-based|One-based),popup(Clip index|Clip and warn|Generate error),checkbox
      mask Display:
      | disp(['Permute\n' modeVal]);
      | port_label('input',1,'A');
      | port_label('input',2,'P');
  Reciprocal Condition : Subsystem
      mask Type: Reciprocal Condition
      mask Description: Estimates the reciprocal of the condition of a square input matrix in the 1-norm.  If input is well conditioned, the output is near 1.0.  If input is badly conditioned, output is near 0.0.
      mask Help: eval('blocksethelp');
      mask Display: disp('RCond')
  Submatrix : S-Function  FunctionName=sdspsubmtrx  Parameters=ColSpan, ColStartMode, ColStartIndex, ColEndMode, ColEndIndex, RowSpan, RowStartMode, RowStartIndex, RowEndMode, RowEndIndex  EnableBusSupport=off  mask(Submatrix){RowSpan=Range of rows, RowStartMode=First, RowStartIndex=1, RowEndMode=Last, RowEndIndex=1, ColSpan=Range of columns, ColStartMode=First, ColStartIndex=1, ColEndMode=Last, ColEndIndex=1}
      mask prompts: RowSpan "Row span:"; RowStartMode "Starting row:"; RowStartIndex "Starting row index:"; RowEndMode "Ending row:"; RowEndIndex "Ending row index:"; ColSpan "Column span:"; ColStartMode "Starting column:"; ColStartIndex "Starting column index:"; ColEndMode "Ending column:"; ColEndIndex "Ending column index:"
      mask help:
      | Return selected portion of input matrix.  1-D input signals are treated as 2-D column vectors.  The output is always 2-D.
      |
      | This block performs 1-based indexing.
      mask init:
      | [x1,y1,xc,yc,xi,yi] = dspblksubmatrix('icon');
      mask Help: eval('blocksethelp');
      mask StyleString: popup(All rows|One row|Range of rows),popup(First|Index|Offset from last|Last|Offset from middle|Middle),edit,popup(Index|Offset from last|Last|Offset from middle|Middle),edit,popup(All columns|One column|Range of columns),popup(First|Index|Offset from last|Last|Offset from middle|Middle),edit,popup(Index|Offset from last|Last|Offset from middle|Middle),edit
      mask CallbackString: dspblksubmatrix|dspblksubmatrix||dspblksubmatrix||dspblksubmatrix|dspblksubmatrix||dspblksubmatrix|
      mask Display: plot(x1,y1,xc,yc,xi,yi);
  Toeplitz : S-Function  FunctionName=sdspmtoep2  Parameters=Symmetric,1,overflowFlag+1  EnableBusSupport=off  mask(Toeplitz){Symmetric=on, overflowFlag=on}
      mask prompts: overflowFlag "Saturate on integer overflow"
      mask help: Generate a symmetric or asymmetric Toeplitz matrix. If Symmetric is selected, a symmetric (or Hermitian) Toeplitz matrix is generated. If Symmetric is not selected, an asymmetric Toeplitz matrix is generated. The columns and rows are specified by the first and second inputs, respectively. The first matrix element is inherited from the column.
      mask init:
      | if (Symmetric==1)
      |   % Do not display anything on ports for this case
      |   p1 = 1; L1 = '';
      |   p2 = 1;  L2 = '';
      |   % Icon display is diagonal matrix picture
      |   horiz_offset = 0.1;
      |   xm=horiz_offset + .8*[0.25 0.1625 0.1625 0.25 NaN 0.7875 0.8875 0.8875 0.7875 NaN 0.25 0.75 NaN 0.4125 0.75 NaN 0.5875 0.75 NaN 0.25 0.5875 NaN 0.25 0.4125];
      |   ym=[.9 .9 .1 .1 NaN .9 .9 .1 .1 NaN .8 .2 NaN .8 .4 NaN .8 .6 NaN .6 .2 NaN .4 .2];
      | else
      |   p1 = 1;  L1 = 'Toep Col';
      |   p2 = 2;  L2 = 'Toep Row';
      |   % Icon display is blank
      |   xm = 0;
      |   ym = 0;
      | end
      mask Help: eval('blocksethelp');
      mask CallbackString:
      | if (strcmp(get_param(gcbh,'Symmetric'),'on'))
      | 	set_param(gcbh,'MaskVisibilities',{'on','on'})
      | else
      | 	set_param(gcbh,'MaskVisibilities',{'on','off'})
      | end|
      mask Display:
      | plot(xm,ym);
      | port_label('input', p1, L1);
      | port_label('input', p2, L2);
  Transpose : Subsystem  mask(Transpose){Hermitian=off, overflowFlag=off}
      mask prompts: overflowFlag "Saturate on integer overflow"
      mask help: Compute the matrix transpose. Vector input signals are treated as [Mx1] matrices. The output is always a matrix.
      mask init:
      | if(Hermitian==1)
      |     str = 'u^H';
      |     set_param([gcb '/Math Function'],'Operator','hermitian');
      |     if (overflowFlag==1)
      |         set_param([gcb '/Math Function'],'SaturateOnIntegerOverflow','on');
      |     else
      |         set_param([gcb '/Math Function'],'SaturateOnIntegerOverflow','off');
      |     end
      | else
      |     str = 'u^T';
      |     set_param([gcb '/Math Function'],'Operator','transpose');
      | end
      mask Help: eval('blocksethelp');
      mask CallbackString:
      | if (strcmp(get_param(gcbh,'Hermitian'),'on'))
      | 	set_param(gcbh,'MaskVisibilities',{'on','on'});
      | else
      | 	set_param(gcbh,'MaskVisibilities',{'on','off'});
      | end|
      mask Display: disp(str,'texmode','on')

== system dspmtrx3/Constant Diagonal Matrix ==
  Constant : Constant  Value=a
  Frame Status Conversion : FrameConversion  OutFrame=Sample-based
  out : Outport  InitialOutput=0
  wires:
  Constant/1 -> Frame Status Conversion/1
  Frame Status Conversion/1 -> out/1

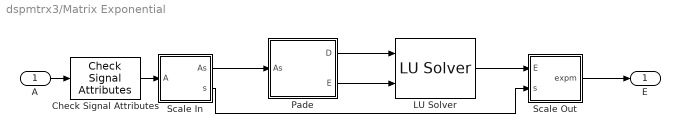
== system dspmtrx3/Matrix Exponential ==
  A : Inport
  Check Signal Attributes : dspsigattribs/Check Signal Attributes  SigAttribCheckMethod=Does not match attributes exactly  Complexity=Ignore  Frame=Ignore  DimsCheckMethod=Is...  Dimensions=Square matrix (2-D)  DatatypeCheckMethod=Is...  DatatypeGeneral=Floating-point  DtypeFloatSpecific=Any floating-point  DtypeFixedSpecific=Any fixed-point  DtypeIntSpecific=Any integer  SampleMode=Ignore
  LU Solver : dspsolvers/LU Solver
  Pade : Subsystem
      mask Display: disp('Pade\nApprox')
  Scale In : Subsystem
  Scale Out : Subsystem
  E : Outport
  wires:
  Check Signal Attributes/1 -> Scale In/1(A)
  A/1 -> Check Signal Attributes/1
  Scale In/1(As) -> Pade/1(As)
  Scale Out/1(expm) -> E/1
  Scale In/2(s) -> Scale Out/2(s)
  Pade/2(E) -> LU Solver/2
  Pade/1(D) -> LU Solver/1
  LU Solver/1 -> Scale Out/1(E)

== system dspmtrx3/Matrix Square ==
  In : Inport
  Math Function : Math  Operator=hermitian
  Product : Product  Multiplication=Matrix(*)  OutMin=OutMin  OutMax=OutMax  OutDataTypeStr=OutDataTypeStr  InputSameDT=on
  Out : Outport
  wires:
  Math Function/1 -> Product/1
  Product/1 -> Out/1
  In/1 -> Math Function/1, Product/2
